simulink library "aausat3_lib"  (Simulink 8.3)
settings: Solver=ode45  StartTime=0.0  StopTime=10.0  RelTol=1e-3
undefined symbols (not defined in the file or in its folder): A_wire_mt, albedo_wrapper, alpha_0_mt, bias_gyro, bias_mag, bias_sun, Cd, coil_dim, Dim, f_sample, G, heading_gyro, heading_mag, M_earth, M_moon, M_sun, magnitude, n_mt, noise_gyro, noise_mag, noise_sun, nr_sample_sun, otoquest, otoquest_with_pro, q_method, qmethod, redfac, refldata, s_freq_gyro, s_freq_mag, s_freq_sun, sigma_0_mt, solar_absorb_coeff, solar_m_flux, SVD_method, T_0_mt, theta_e, tilt_gyro, tilt_mag, Ts
undefined symbols (not defined in the file): Actuator_Duty_Cycle_coil, Actuator_Frequency_coil, Dimensions_coil, mean_refl, Number_of_Windings_coil, rho, sim_par, svd_weigth, Wire_Cross_Sectional_Area_coil, Wire_Resistivity_Base_Temperature_coil, Wire_Resistivity_coil, Wire_Resistivity_Temperature_Coefficient_coil
libraries: aausat3_lib x118, simulink_extras x3
(part 2 of 4)

== system aausat3_lib/ADS/q-method (AAUSAT3) ==
  Sun_S : Inport  SampleTime=1
  Mag_S : Inport  Port=2  SampleTime=1
  Sun_I : Inport  Port=3  SampleTime=1
  Mag_I : Inport  Port=4  SampleTime=1
  Mux : Mux  Inputs=5
  To unit vector{,1..3} (4 alike) : aausat3_lib/Math Utilities/Vector operations/To unit vector  SystemSampleTime=-1
  Weights : Constant  Value=weigth_a
  qmethod.m : MATLABFcn  MATLABFcn=q_method([u(1) u(4);u(2) u(5);u(3) u(6)] , [u(7) u(10);u(8) u(11); u(9) u(12)], [u(13);u(14)])  OutputDimensions=4  Output1D=off
  q(I->S) : Outport  PortDimensions=4
  wires:
  Sun_I/1 -> To unit vector2/1
  Mux/1 -> qmethod.m/1
  To unit vector/1 -> Mux/1
  To unit vector2/1 -> Mux/3
  Sun_S/1 -> To unit vector/1
  Mag_I/1 -> To unit vector3/1
  To unit vector3/1 -> Mux/4
  To unit vector1/1 -> Mux/2
  Mag_S/1 -> To unit vector1/1
  Weights/1 -> Mux/5
  qmethod.m/1 -> q(I->S)/1

== system aausat3_lib/ADS/svd-method (AAUSAT3) ==
  Sun_S : Inport  SampleTime=1
  Mag_S : Inport  Port=2  SampleTime=1
  Sun_I : Inport  Port=3  SampleTime=1
  Mag_I : Inport  Port=4  SampleTime=1
  Enable : EnablePort
  Demux : Demux  Outputs=5
  Mux : Mux  Inputs=5
  Mux1 : Mux
  To unit vector{,1..3} (4 alike) : aausat3_lib/Math Utilities/Vector operations/To unit vector  SystemSampleTime=-1
  Weights : Constant  Value=weigth_a
  svd_method.m : MATLABFcn  MATLABFcn=SVD_method(u(13),[u(7);u(8);u(9)],[u(1);u(2);u(3)],u(14),[u(10);u(11);u(12)],[u(4);u(5);u(6)],0)  OutputDimensions=5  Output1D=off  SampleTime=1/f_sample
  q(I->S) : Outport  PortDimensions=4
  err : Outport  Port=2
  wires:
  Demux/5 -> err/1
  Mux1/1 -> q(I->S)/1
  svd_method.m/1 -> Demux/1
  Demux/4 -> Mux1/4
  Demux/3 -> Mux1/3
  Demux/2 -> Mux1/2
  Demux/1 -> Mux1/1
  Sun_I/1 -> To unit vector2/1
  Mux/1 -> svd_method.m/1
  To unit vector/1 -> Mux/1
  To unit vector2/1 -> Mux/3
  Sun_S/1 -> To unit vector/1
  Mag_I/1 -> To unit vector3/1
  To unit vector3/1 -> Mux/4
  To unit vector1/1 -> Mux/2
  Mag_S/1 -> To unit vector1/1
  Weights/1 -> Mux/5

== system aausat3_lib/Actuator Emulation/Magnetorquer ==
  note: m_{mt_{vec}}
  note: m_{mt}
  note: i_{mt}
  note: R_{mt}(T)
  v_mt : Inport
  coil normal : Inport  Port=2
  B(s) : Inport  Port=3
  T : Inport  Port=4
  Abs : Abs
  Area : Constant  Value=coil_dim(1)*coil_dim(2)
  Cross Product : aausat3_lib/Math Utilities/Vector operations/Cross Product
  Prodct1 : Product  Inputs=*/  RndMeth=Zero
  Prodct5 : Product  Inputs=*/  RndMeth=Zero
  Product : Product  Inputs=3  RndMeth=Zero
  Product1 : Product  Inputs=3  RndMeth=Zero
  Product2 : Product  RndMeth=Zero
  Product3 : Product  Inputs=3  RndMeth=Zero
  Product5 : Product  RndMeth=Zero
  Resistivity : Constant  Value=sigma_0_mt
  Resistivity base temperature : Constant  Value=T_0_mt
  Resistivity temperature coefficient : Constant  Value=alpha_0_mt
  Sum : Sum  Inputs=|+-
  Sum1 : Sum  Inputs=|++
  Windings : Constant  Value=n_mt
  Windings1 : Constant  Value=n_mt
  Wire cross sectional area : Constant  Value=A_wire_mt
  wire  circumference : Constant  Value=2*coil_dim(1)+2*coil_dim(2)
  N_mt(s) : Outport
  P_mt : Outport  Port=2
  m_mt_max : Outport  Port=3
  wires:
  Cross Product/1 -> N_mt(s)/1
  Product2/1 -> m_mt_max/1, Cross Product/1
  Product/1 -> Product2/2
  Area/1 -> Product/2
  Windings/1 -> Product/1
  Prodct1/1 -> Product/3, Product5/1
  coil normal/1 -> Product2/1
  Resistivity base temperature/1 -> Sum/2
  T/1 -> Sum/1
  Resistivity temperature coefficient/1 -> Product1/2
  Sum/1 -> Product1/1
  Resistivity/1 -> Product1/3, Sum1/2
  Product1/1 -> Sum1/1
  Sum1/1 -> Product3/1
  wire  circumference/1 -> Product3/2
  Windings1/1 -> Product3/3
  Product3/1 -> Prodct5/1
  Wire cross sectional area/1 -> Prodct5/2
  Prodct5/1 -> Prodct1/2
  B(s)/1 -> Cross Product/2
  v_mt/1 -> Prodct1/1, Product5/2
  Product5/1 -> Abs/1
  Abs/1 -> P_mt/1

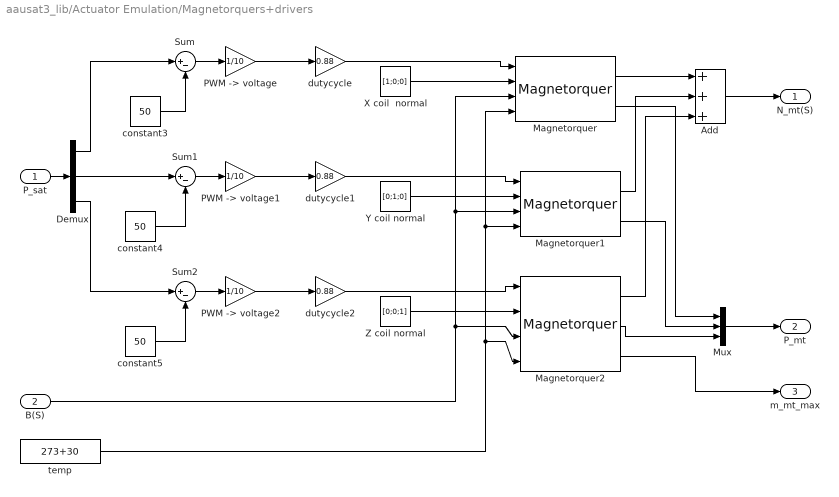
== system aausat3_lib/Actuator Emulation/Magnetorquers+drivers ==
  P_sat : Inport
  B(S) : Inport  Port=2
  Add : Sum  Inputs=+++
  Demux : Demux  Outputs=3
  Magnetorquer : aausat3_lib/Actuator Emulation/Magnetorquer  SystemSampleTime=-1  coil_dim=coil_dim  n_mt=n_mt  A_wire_mt=A_wire_mt  sigma_0_mt=sigma_0_mt  alpha_0_mt=alpha_0_mt  T_0_mt=T_0_mt
  Magnetorquer1 : aausat3_lib/Actuator Emulation/Magnetorquer  SystemSampleTime=-1  coil_dim=coil_dim  n_mt=n_mt  A_wire_mt=A_wire_mt  sigma_0_mt=sigma_0_mt  alpha_0_mt=alpha_0_mt  T_0_mt=T_0_mt
  Magnetorquer2 : aausat3_lib/Actuator Emulation/Magnetorquer  SystemSampleTime=-1  coil_dim=coil_dim  n_mt=n_mt  A_wire_mt=A_wire_mt  sigma_0_mt=sigma_0_mt  alpha_0_mt=alpha_0_mt  T_0_mt=T_0_mt
  Mux : Mux  Inputs=3
  "PWM -> voltage" : Gain  Gain=1/10
  "PWM -> voltage1" : Gain  Gain=1/10
  "PWM -> voltage2" : Gain  Gain=1/10
  Sum : Sum  Inputs=|+-
  Sum1 : Sum  Inputs=|+-
  Sum2 : Sum  Inputs=|+-
  X coil  normal : Constant  Value=[1;0;0]
  Y coil normal : Constant  Value=[0;1;0]
  Z coil normal : Constant  Value=[0;0;1]
  constant3 : Constant  Value=50
  constant4 : Constant  Value=50
  constant5 : Constant  Value=50
  dutycycle : Gain  Gain=0.88
  dutycycle1 : Gain  Gain=0.88
  dutycycle2 : Gain  Gain=0.88
  temp : Constant  Value=273+30
  N_mt(S) : Outport  PortDimensions=3
  P_mt : Outport  Port=2  PortDimensions=3
  m_mt_max : Outport  Port=3
  wires:
  Magnetorquer2/3 -> m_mt_max/1
  "PWM -> voltage2"/1 -> dutycycle2/1
  "PWM -> voltage1"/1 -> dutycycle1/1
  "PWM -> voltage"/1 -> dutycycle/1
  temp/1 -> Magnetorquer/4, Magnetorquer1/4, Magnetorquer2/4
  B(S)/1 -> Magnetorquer/3, Magnetorquer1/3, Magnetorquer2/3
  Z coil normal/1 -> Magnetorquer2/2
  Y coil normal/1 -> Magnetorquer1/2
  Magnetorquer2/1 -> Add/3
  Magnetorquer1/1 -> Add/2
  Magnetorquer/1 -> Add/1
  X coil  normal/1 -> Magnetorquer/2
  Add/1 -> N_mt(S)/1
  Magnetorquer/2 -> Mux/1
  Magnetorquer1/2 -> Mux/2
  Magnetorquer2/2 -> Mux/3
  Mux/1 -> P_mt/1
  dutycycle/1 -> Magnetorquer/1
  dutycycle1/1 -> Magnetorquer1/1
  dutycycle2/1 -> Magnetorquer2/1
  P_sat/1 -> Demux/1
  Demux/2 -> Sum1/1
  Demux/1 -> Sum/1
  Demux/3 -> Sum2/1
  Sum/1 -> "PWM -> voltage"/1
  constant3/1 -> Sum/2
  Sum1/1 -> "PWM -> voltage1"/1
  constant4/1 -> Sum1/2
  Sum2/1 -> "PWM -> voltage2"/1
  constant5/1 -> Sum2/2

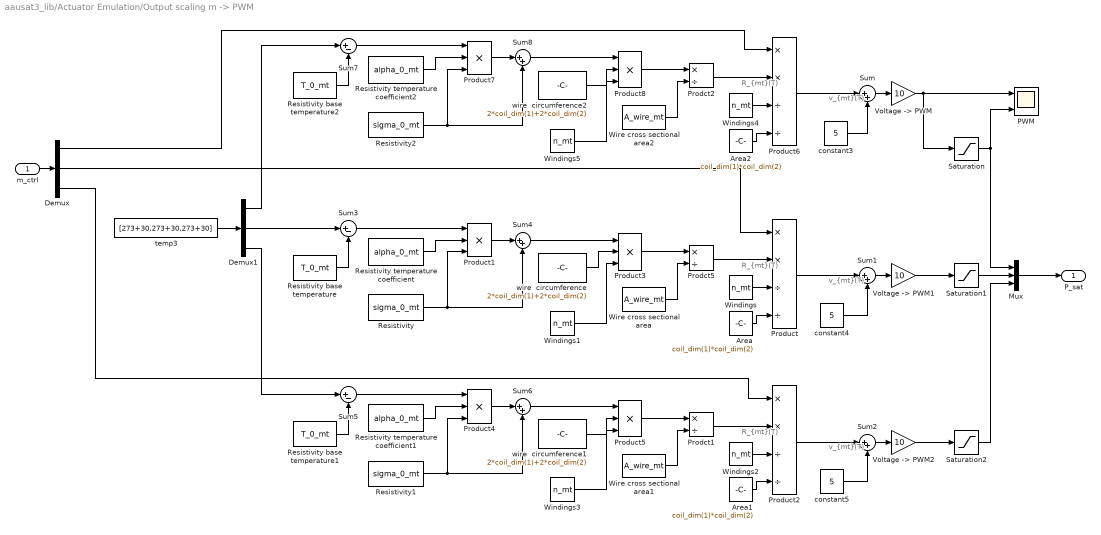
== system aausat3_lib/Actuator Emulation/Output scaling m -> PWM ==
  note: R_{mt}(T)
  note: R_{mt}(T)
  note: R_{mt}(T)
  note: v_{mt}(T)
  note: v_{mt}(T)
  note: v_{mt}(T)
  m_ctrl : Inport
  Area : Constant  Value=coil_dim(1)*coil_dim(2)
  Area1 : Constant  Value=coil_dim(1)*coil_dim(2)
  Area2 : Constant  Value=coil_dim(1)*coil_dim(2)
  Demux : Demux  Outputs=3
  Demux1 : Demux  Outputs=3
  Mux : Mux  Inputs=3
  PWM : Scope  NumInputPorts=2
      settings: TimeRange=5000  YMin=37.5~37.5  YMax=67.5~62.5  SaveName=ScopeData4  SampleInput=on
  Prodct1 : Product  Inputs=*/  RndMeth=Zero
  Prodct2 : Product  Inputs=*/  RndMeth=Zero
  Prodct5 : Product  Inputs=*/  RndMeth=Zero
  Product : Product  Inputs=**//  RndMeth=Zero
  Product{1,3..5,7..8} (6 alike) : Product  Inputs=3  RndMeth=Zero
  Product2 : Product  Inputs=**//  RndMeth=Zero
  Product6 : Product  Inputs=**//  RndMeth=Zero
  Resistivity : Constant  Value=sigma_0_mt
  Resistivity base temperature : Constant  Value=T_0_mt
  Resistivity base temperature1 : Constant  Value=T_0_mt
  Resistivity base temperature2 : Constant  Value=T_0_mt
  Resistivity temperature coefficient : Constant  Value=alpha_0_mt
  Resistivity temperature coefficient1 : Constant  Value=alpha_0_mt
  Resistivity temperature coefficient2 : Constant  Value=alpha_0_mt
  Resistivity1 : Constant  Value=sigma_0_mt
  Resistivity2 : Constant  Value=sigma_0_mt
  Saturation : Saturate  UpperLimit=PWM_max  LowerLimit=PWM_min
  Saturation1 : Saturate  UpperLimit=PWM_max  LowerLimit=PWM_min
  Saturation2 : Saturate  UpperLimit=PWM_max  LowerLimit=PWM_min
  Sum{,1..2,4,6,8} (6 alike) : Sum  Inputs=|++
  Sum3 : Sum  Inputs=|+-
  Sum5 : Sum  Inputs=|+-
  Sum7 : Sum  Inputs=|+-
  "Voltage -> PWM" : Gain  Gain=10
  "Voltage -> PWM1" : Gain  Gain=10
  "Voltage -> PWM2" : Gain  Gain=10
  Windings{,1..5} (6 alike) : Constant  Value=n_mt
  Wire cross sectional area : Constant  Value=A_wire_mt
  Wire cross sectional area1 : Constant  Value=A_wire_mt
  Wire cross sectional area2 : Constant  Value=A_wire_mt
  constant3 : Constant  Value=5
  constant4 : Constant  Value=5
  constant5 : Constant  Value=5
  temp3 : Constant  Value=[273+30,273+30,273+30]
  wire  circumference : Constant  Value=2*coil_dim(1)+2*coil_dim(2)
  wire  circumference1 : Constant  Value=2*coil_dim(1)+2*coil_dim(2)
  wire  circumference2 : Constant  Value=2*coil_dim(1)+2*coil_dim(2)
  P_sat : Outport  PortDimensions=3
  wires:
  Prodct2/1 -> Product6/2
  Prodct5/1 -> Product/2
  Prodct1/1 -> Product2/2
  Resistivity base temperature2/1 -> Sum7/2
  Resistivity temperature coefficient2/1 -> Product7/2
  Sum7/1 -> Product7/1
  Resistivity2/1 -> Product7/3, Sum8/2
  Product7/1 -> Sum8/1
  Sum8/1 -> Product8/1
  wire  circumference2/1 -> Product8/2
  Windings5/1 -> Product8/3
  Product8/1 -> Prodct2/1
  Wire cross sectional area2/1 -> Prodct2/2
  Demux1/1 -> Sum7/1
  Resistivity base temperature/1 -> Sum3/2
  Resistivity temperature coefficient/1 -> Product1/2
  Sum3/1 -> Product1/1
  Resistivity/1 -> Product1/3, Sum4/2
  Product1/1 -> Sum4/1
  Sum4/1 -> Product3/1
  wire  circumference/1 -> Product3/2
  Windings1/1 -> Product3/3
  Product3/1 -> Prodct5/1
  Wire cross sectional area/1 -> Prodct5/2
  Demux1/2 -> Sum3/1
  Demux1/3 -> Sum5/1
  Resistivity base temperature1/1 -> Sum5/2
  Resistivity temperature coefficient1/1 -> Product4/2
  Sum5/1 -> Product4/1
  Resistivity1/1 -> Product4/3, Sum6/2
  Product4/1 -> Sum6/1
  Sum6/1 -> Product5/1
  wire  circumference1/1 -> Product5/2
  Windings3/1 -> Product5/3
  Product5/1 -> Prodct1/1
  Wire cross sectional area1/1 -> Prodct1/2
  constant5/1 -> Sum2/2
  constant4/1 -> Sum1/2
  constant3/1 -> Sum/2
  m_ctrl/1 -> Demux/1
  Mux/1 -> P_sat/1
  Saturation/1 -> PWM/2, Mux/1
  Saturation1/1 -> Mux/2
  Saturation2/1 -> Mux/3
  Sum/1 -> "Voltage -> PWM"/1
  Sum1/1 -> "Voltage -> PWM1"/1
  Sum2/1 -> "Voltage -> PWM2"/1
  temp3/1 -> Demux1/1
  Windings/1 -> Product/3
  Area/1 -> Product/4
  Windings2/1 -> Product2/3
  Area1/1 -> Product2/4
  Windings4/1 -> Product6/3
  Area2/1 -> Product6/4
  "Voltage -> PWM"/1 -> PWM/1, Saturation/1
  "Voltage -> PWM1"/1 -> Saturation1/1
  "Voltage -> PWM2"/1 -> Saturation2/1
  Demux/1 -> Product6/1
  Demux/2 -> Product/1
  Demux/3 -> Product2/1
  Product6/1 -> Sum/1
  Product/1 -> Sum1/1
  Product2/1 -> Sum2/1

== system aausat3_lib/Actuator Emulation/Permanent Magnet ==
  Attitude q(I->S) : Inport
  Magnetic field B(I) : Inport  Port=2
  Enable : EnablePort
  Cross Product : aausat3_lib/Math Utilities/Vector operations/Cross Product  SystemSampleTime=-1
  Magnetic dipole moment : Constant  Value=[0,0,mag_moment]
  Vector rotation by q : Subsystem
  N_mpmag(S) : Outport
  wires:
  Magnetic dipole moment/1 -> Cross Product/1
  Vector rotation by q/1(q'Vq) -> Cross Product/2
  Cross Product/1 -> N_mpmag(S)/1
  Attitude q(I->S)/1 -> Vector rotation by q/1(q)
  Magnetic field B(I)/1 -> Vector rotation by q/2(V)

== system aausat3_lib/Disturbances/Atmospheric ==
  q(I->S) : Inport
  V_sc(I) : Inport  Port=2
  R_com(S) : Inport  Port=3
  inclination : Inport  Port=4
  r_pos : Inport  Port=5
  jd : Inport  Port=6
  Enable : EnablePort
  C_D1 : Constant  Value=Cd
  Demux : Demux  Outputs=6
  Density7 : Subsystem
  MATLAB Function : MATLAB Function  TreatAsAtomicUnit=on
  Mux : Mux  Inputs=6
  Mux1 : Mux  Inputs=3
  Mux2 : Mux  Inputs=3
  N_atm(S) : Outport
  F_atm(I) : Outport  Port=2
  wires:
  Mux/1 -> MATLAB Function/1(input)
  MATLAB Function/1(out) -> Demux/1
  Demux/3 -> Mux1/3
  Demux/2 -> Mux1/2
  Demux/1 -> Mux1/1
  Demux/6 -> Mux2/3
  Demux/5 -> Mux2/2
  Demux/4 -> Mux2/1
  Mux2/1 -> F_atm(I)/1
  Mux1/1 -> N_atm(S)/1
  q(I->S)/1 -> Mux/6
  V_sc(I)/1 -> Mux/4
  C_D1/1 -> Mux/2
  jd/1 -> Density7/3(jd)
  inclination/1 -> Density7/1(i)
  r_pos/1 -> Density7/2(r), Mux/5
  Density7/1(rho) -> Mux/1
  R_com(S)/1 -> Mux/3  "Center of Mass"

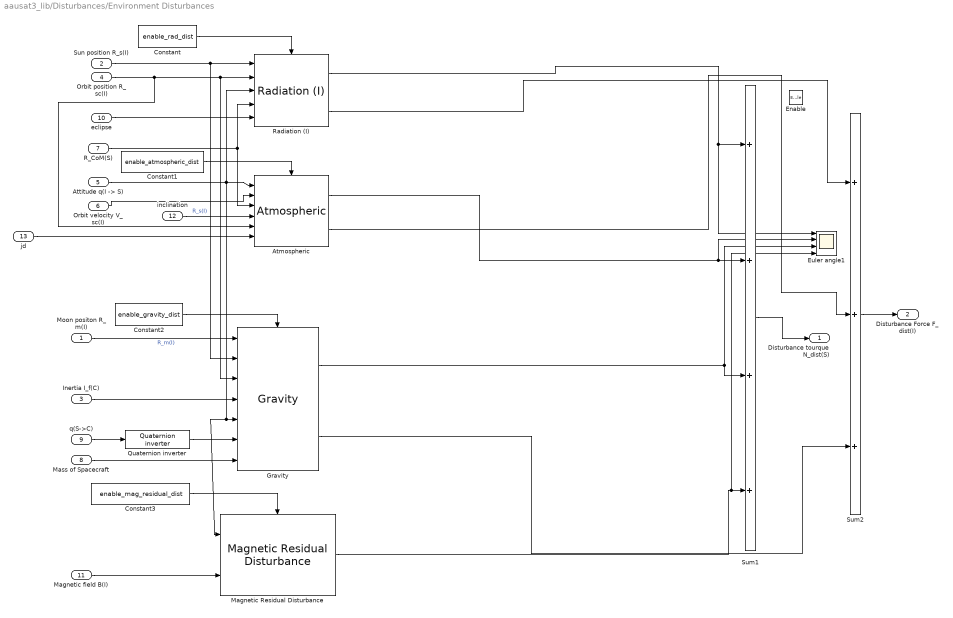
== system aausat3_lib/Disturbances/Environment Disturbances ==
  Moon positon R_m(I) : Inport
  Sun position R_s(I) : Inport  Port=2
  Inertia I_f(C) : Inport  Port=3
  Orbit position R_sc(I) : Inport  Port=4
  "Attitude q(I -> S)" : Inport  Port=5
  Orbit velocity V_sc(I) : Inport  Port=6
  R_CoM(S) : Inport  Port=7
  Mass of Spacecraft : Inport  Port=8
  q(S->C) : Inport  Port=9
  eclipse : Inport  Port=10
  Magnetic field B(I) : Inport  Port=11
  inclination : Inport  Port=12
  jd : Inport  Port=13
  Enable : EnablePort
  Atmospheric : aausat3_lib/Disturbances/Atmospheric  Cd=Cd  rho=rho
  Constant : Constant  Value=enable_rad_dist
  Constant1 : Constant  Value=enable_atmospheric_dist
  Constant2 : Constant  Value=enable_gravity_dist
  Constant3 : Constant  Value=enable_mag_residual_dist
  Euler angle1 : Scope  NumInputPorts=4
      settings: TimeRange=5000  YMin=-2e-08~-4e-07~-1.5e-08~-4e-08  YMax=2e-08~4e-07~1.5e-08~4e-08  SaveName=dist_sep  SampleInput=on
  Gravity : aausat3_lib/Disturbances/Gravity  G=G  M_sun=M_sun  M_moon=M_moon  M_earth=M_earth  enable_moon_G=on  enable_sun_G=on  enable_zharm_earth=on  enable_gravity_torque=on
  Magnetic Residual Disturbance : aausat3_lib/Disturbances/Magnetic Residual Disturbance  mag_moment=0.00033
  Quaternion inverter : aausat3_lib/Math Utilities/Quaternion operations/Quaternion inverter
  Radiation (I) : aausat3_lib/Disturbances/Radiation (I)  Dim=Dim  solar_m_flux=solar_m_flux  solar_absorb_coeff=solar_absorb_coeff
  Sum1 : Sum  Inputs=++++  SaturateOnIntegerOverflow=on
  Sum2 : Sum  Inputs=+++  SaturateOnIntegerOverflow=on
  Disturbance tourque N_dist(S) : Outport
  Disturbance Force F_dist(I) : Outport  Port=2
  wires:
  jd/1 -> Atmospheric/6
  inclination/1 -> Atmospheric/4
  Sum2/1 -> Disturbance Force F_dist(I)/1
  Radiation (I)/1 -> Euler angle1/1, Sum1/1
  Atmospheric/1 -> Euler angle1/2, Sum1/2
  Gravity/1 -> Euler angle1/3, Sum1/3
  Magnetic Residual Disturbance/1 -> Euler angle1/4, Sum1/4
  Atmospheric/2 -> Sum2/2
  Inertia I_f(C)/1 -> Gravity/4
  eclipse/1 -> Radiation (I)/5
  Sum1/1 -> Disturbance tourque N_dist(S)/1
  Gravity/2 -> Sum2/3
  Radiation (I)/2 -> Sum2/1
  Orbit velocity V_sc(I)/1 -> Atmospheric/2
  Orbit position R_sc(I)/1 -> Radiation (I)/2, Gravity/3, Atmospheric/5
  "Attitude q(I -> S)"/1 -> Radiation (I)/3, Atmospheric/1, Gravity/5, Magnetic Residual Disturbance/1
  Sun position R_s(I)/1 -> Radiation (I)/1, Gravity/2  "R_s(I)"
  Moon positon R_m(I)/1 -> Gravity/1  "R_m(I)"
  Mass of Spacecraft/1 -> Gravity/7
  Quaternion inverter/1 -> Gravity/6
  q(S->C)/1 -> Quaternion inverter/1
  R_CoM(S)/1 -> Radiation (I)/4, Atmospheric/3
  Constant/1 -> Radiation (I)/Enable
  Constant2/1 -> Gravity/Enable
  Constant1/1 -> Atmospheric/Enable
  Constant3/1 -> Magnetic Residual Disturbance/Enable
  Magnetic field B(I)/1 -> Magnetic Residual Disturbance/2

== system aausat3_lib/Disturbances/Gravity ==
  R_m(I) : Inport
  R_s(I) : Inport  Port=2
  R_sc(I) : Inport  Port=3
  I(C) : Inport  Port=4
  "q(I -> S)" : Inport  Port=5
  q(C->S) : Inport  Port=6
  M_sat : Inport  Port=7
  Enable : EnablePort
  Constant : Constant  Value=enable_moon_G
  Constant1 : Constant  Value=enable_sun_G
  Constant2 : Constant  Value=enable_zharm_earth
  Constant3 : Constant  Value=enable_gravity_torque
  Gravity Gradient Torque : aausat3_lib/Disturbances/Gravity Gradient Torque  G=G  M_earth=M_earth
  Gravity Moon : aausat3_lib/Disturbances/Gravity Moon  G=G  M_moon=M_moon
  Gravity Sun : aausat3_lib/Disturbances/Gravity Sun  G=G  M_sun=M_sun
  Sum : Sum  Inputs=++++  SaturateOnIntegerOverflow=on
  Sum1 : Sum  Inputs=|+-  SaturateOnIntegerOverflow=on
  Sum2 : Sum  Inputs=|+-  SaturateOnIntegerOverflow=on
  Sum3 : Sum  Inputs=++++  SaturateOnIntegerOverflow=on
  Zonal Harmonics  Earth : aausat3_lib/Disturbances/Zonal Harmonics  Earth
  N_gr(S) : Outport
  F_gr(I) : Outport  Port=2
  wires:
  Zonal Harmonics  Earth/2 -> Sum3/3
  Gravity Sun/2 -> Sum3/2
  Gravity Moon/2 -> Sum3/1
  Sum3/1 -> N_gr(S)/1
  I(C)/1 -> Zonal Harmonics  Earth/3, Gravity Sun/2, Gravity Moon/2, Gravity Gradient Torque/2
  q(C->S)/1 -> Zonal Harmonics  Earth/4, Gravity Sun/3, Gravity Moon/3, Gravity Gradient Torque/3
  "q(I -> S)"/1 -> Zonal Harmonics  Earth/5, Gravity Gradient Torque/4, Gravity Sun/4, Gravity Moon/4
  M_sat/1 -> Gravity Sun/1, Zonal Harmonics  Earth/1, Gravity Moon/1, Gravity Gradient Torque/5
  Sum/1 -> F_gr(I)/1
  Zonal Harmonics  Earth/1 -> Sum/3
  R_m(I)/1 -> Sum1/1
  R_s(I)/1 -> Sum2/1
  Gravity Moon/1 -> Sum/1
  Gravity Sun/1 -> Sum/2
  Constant3/1 -> Gravity Gradient Torque/Enable
  Constant2/1 -> Zonal Harmonics  Earth/Enable
  Constant1/1 -> Gravity Sun/Enable
  Constant/1 -> Gravity Moon/Enable
  R_sc(I)/1 -> Sum1/2, Sum2/2, Zonal Harmonics  Earth/2, Gravity Gradient Torque/1
  Sum2/1 -> Gravity Sun/5
  Sum1/1 -> Gravity Moon/5
  Gravity Gradient Torque/1 -> Sum3/4
  Gravity Gradient Torque/2 -> Sum/4

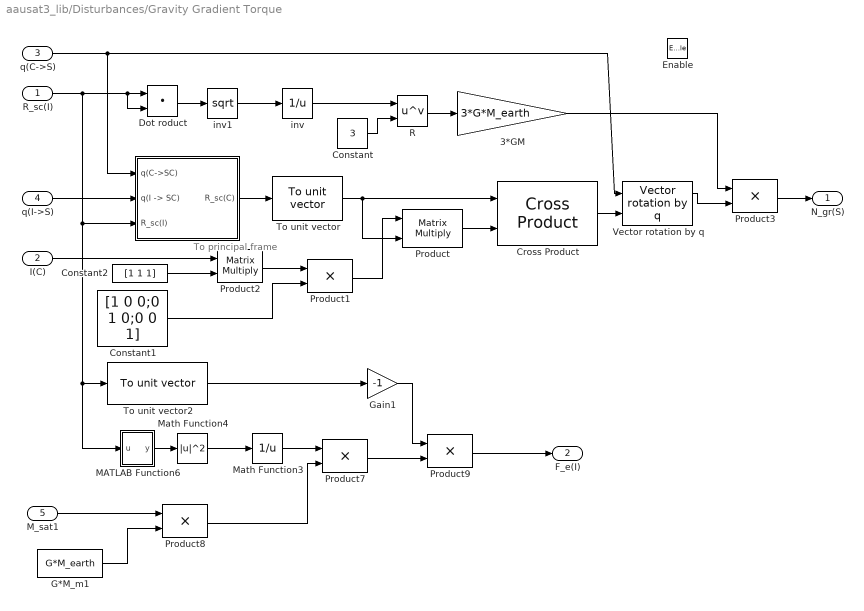
== system aausat3_lib/Disturbances/Gravity Gradient Torque ==
  note: To principal frame
  R_sc(I) : Inport
  I(C) : Inport  Port=2
  q(C->S) : Inport  Port=3
  q(I->S) : Inport  Port=4
  M_sat1 : Inport  Port=5
  Enable : EnablePort
  " " : Subsystem
  3*GM : Gain  Gain=3*G*M_earth  SaturateOnIntegerOverflow=on  OutDataTypeStr=Inherit: Same as input  ParamDataTypeStr=Inherit: Same as input
  Constant : Constant  Value=3
  Constant1 : Constant  Value=[1 0 0;0 1 0;0 0 1]
  Constant2 : Constant  Value=[1 1 1]  VectorParams1D=off
  Cross Product : aausat3_lib/Math Utilities/Vector operations/Cross Product
  Dot roduct : DotProduct  InputSameDT=on  OutDataTypeStr=Inherit: Inherit via internal rule
  G*M_m1 : Constant  Value=G*M_earth
  Gain1 : Gain  Gain=-1  SaturateOnIntegerOverflow=on  OutDataTypeStr=Inherit: Same as input  ParamDataTypeStr=Inherit: Same as input
  MATLAB Function6 : MATLAB Function  TreatAsAtomicUnit=on
  Math Function3 : Math  Operator=reciprocal  SaturateOnIntegerOverflow=on
  Math Function4 : Math  Operator=magnitude^2  SaturateOnIntegerOverflow=on
  Product : Product  Multiplication=Matrix(*)  SaturateOnIntegerOverflow=on  OutDataTypeStr=Inherit: Same as first input
  Product{1,3,7..9} (5 alike) : Product  SaturateOnIntegerOverflow=on  OutDataTypeStr=Inherit: Same as first input
  Product2 : Product  Multiplication=Matrix(*)  SaturateOnIntegerOverflow=on  OutDataTypeStr=Inherit: Same as first input
  R : Math  Operator=pow  SaturateOnIntegerOverflow=on
  To unit vector : aausat3_lib/Math Utilities/Vector operations/To unit vector
  To unit vector2 : aausat3_lib/Math Utilities/Vector operations/To unit vector
  Vector rotation by q : aausat3_lib/Math Utilities/Quaternion operations/Vector rotation by q
  inv : Math  Operator=reciprocal  SaturateOnIntegerOverflow=on
  inv1 : Math  Operator=sqrt  SaturateOnIntegerOverflow=on
  N_gr(S) : Outport
  F_e(I) : Outport  Port=2
  wires:
  MATLAB Function6/1(y) -> Math Function4/1
  Cross Product/1 -> Vector rotation by q/2
  Dot roduct/1 -> inv1/1
  Product3/1 -> N_gr(S)/1
  R/1 -> 3*GM/1
  inv/1 -> R/1
  inv1/1 -> inv/1
  Constant/1 -> R/2
  To unit vector/1 -> Product/2, Cross Product/1
  q(C->S)/1 -> " "/1(q(C->SC)), Vector rotation by q/1
  q(I->S)/1 -> " "/2("q(I -> SC)")
  " "/1(R_sc(C)) -> To unit vector/1
  Product1/1 -> Product/1
  Product/1 -> Cross Product/2
  I(C)/1 -> Product2/1
  Constant2/1 -> Product2/2
  Product2/1 -> Product1/1
  Constant1/1 -> Product1/2
  R_sc(I)/1 -> Dot roduct/2, Dot roduct/1, " "/3(R_sc(I)), To unit vector2/1, MATLAB Function6/1(u)
  3*GM/1 -> Product3/1
  Vector rotation by q/1 -> Product3/2
  Math Function4/1 -> Math Function3/1
  M_sat1/1 -> Product8/1
  G*M_m1/1 -> Product8/2
  Math Function3/1 -> Product7/1
  Product8/1 -> Product7/2
  To unit vector2/1 -> Gain1/1
  Product9/1 -> F_e(I)/1
  Gain1/1 -> Product9/1
  Product7/1 -> Product9/2

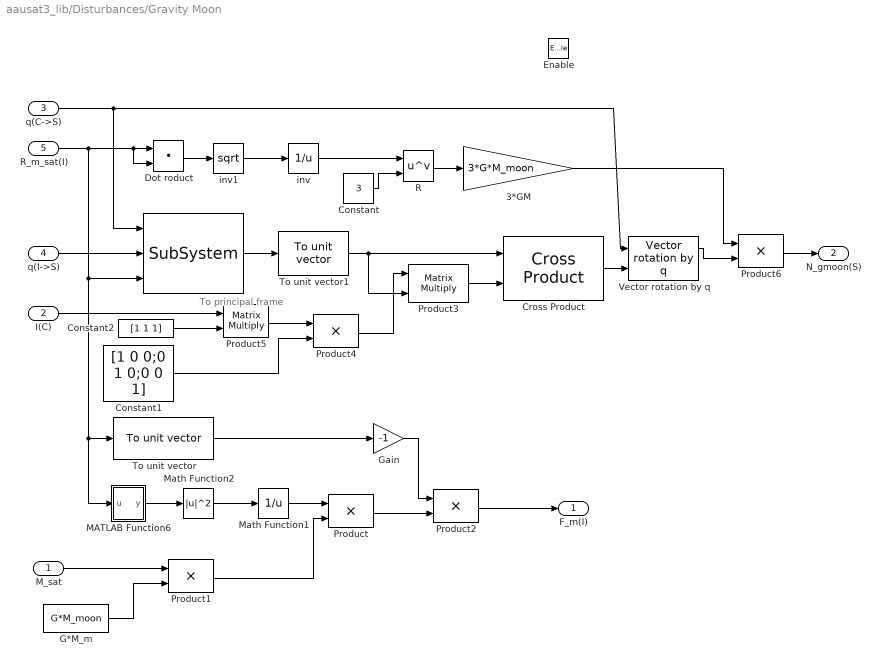
== system aausat3_lib/Disturbances/Gravity Moon ==
  note: To principal frame
  M_sat : Inport
  I(C) : Inport  Port=2
  q(C->S) : Inport  Port=3
  q(I->S) : Inport  Port=4
  R_m_sat(I) : Inport  Port=5
  Enable : EnablePort
  " " : aausat3_lib/Disturbances/Gravity Gradient Torque/ 
  3*GM : Gain  Gain=3*G*M_moon  SaturateOnIntegerOverflow=on  OutDataTypeStr=Inherit: Same as input  ParamDataTypeStr=Inherit: Same as input
  Constant : Constant  Value=3
  Constant1 : Constant  Value=[1 0 0;0 1 0;0 0 1]
  Constant2 : Constant  Value=[1 1 1]  VectorParams1D=off
  Cross Product : aausat3_lib/Math Utilities/Vector operations/Cross Product
  Dot roduct : DotProduct  InputSameDT=on  OutDataTypeStr=Inherit: Inherit via internal rule
  G*M_m : Constant  Value=G*M_moon
  Gain : Gain  Gain=-1  SaturateOnIntegerOverflow=on  OutDataTypeStr=Inherit: Same as input  ParamDataTypeStr=Inherit: Same as input
  MATLAB Function6 : MATLAB Function  TreatAsAtomicUnit=on
  Math Function1 : Math  Operator=reciprocal  SaturateOnIntegerOverflow=on
  Math Function2 : Math  Operator=magnitude^2  SaturateOnIntegerOverflow=on
  Product{,1..2,4,6} (5 alike) : Product  SaturateOnIntegerOverflow=on  OutDataTypeStr=Inherit: Same as first input
  Product3 : Product  Multiplication=Matrix(*)  SaturateOnIntegerOverflow=on  OutDataTypeStr=Inherit: Same as first input
  Product5 : Product  Multiplication=Matrix(*)  SaturateOnIntegerOverflow=on  OutDataTypeStr=Inherit: Same as first input
  R : Math  Operator=pow  SaturateOnIntegerOverflow=on
  To unit vector : aausat3_lib/Math Utilities/Vector operations/To unit vector
  To unit vector1 : aausat3_lib/Math Utilities/Vector operations/To unit vector
  Vector rotation by q : aausat3_lib/Math Utilities/Quaternion operations/Vector rotation by q
  inv : Math  Operator=reciprocal  SaturateOnIntegerOverflow=on
  inv1 : Math  Operator=sqrt  SaturateOnIntegerOverflow=on
  F_m(I) : Outport
  N_gmoon(S) : Outport  Port=2
  wires:
  MATLAB Function6/1(y) -> Math Function2/1
  Math Function2/1 -> Math Function1/1
  M_sat/1 -> Product1/1
  G*M_m/1 -> Product1/2
  Math Function1/1 -> Product/1
  Product1/1 -> Product/2
  To unit vector/1 -> Gain/1
  Product2/1 -> F_m(I)/1
  Gain/1 -> Product2/1
  Product/1 -> Product2/2
  Vector rotation by q/1 -> Product6/2
  3*GM/1 -> Product6/1
  Constant1/1 -> Product4/2
  Product5/1 -> Product4/1
  Constant2/1 -> Product5/2
  I(C)/1 -> Product5/1
  Product3/1 -> Cross Product/2
  Product4/1 -> Product3/1
  " "/1 -> To unit vector1/1
  q(I->S)/1 -> " "/2
  q(C->S)/1 -> Vector rotation by q/1, " "/1
  To unit vector1/1 -> Cross Product/1, Product3/2
  Constant/1 -> R/2
  inv1/1 -> inv/1
  inv/1 -> R/1
  R/1 -> 3*GM/1
  Product6/1 -> N_gmoon(S)/1
  Dot roduct/1 -> inv1/1
  Cross Product/1 -> Vector rotation by q/2
  R_m_sat(I)/1 -> Dot roduct/1, Dot roduct/2, " "/3, To unit vector/1, MATLAB Function6/1(u)

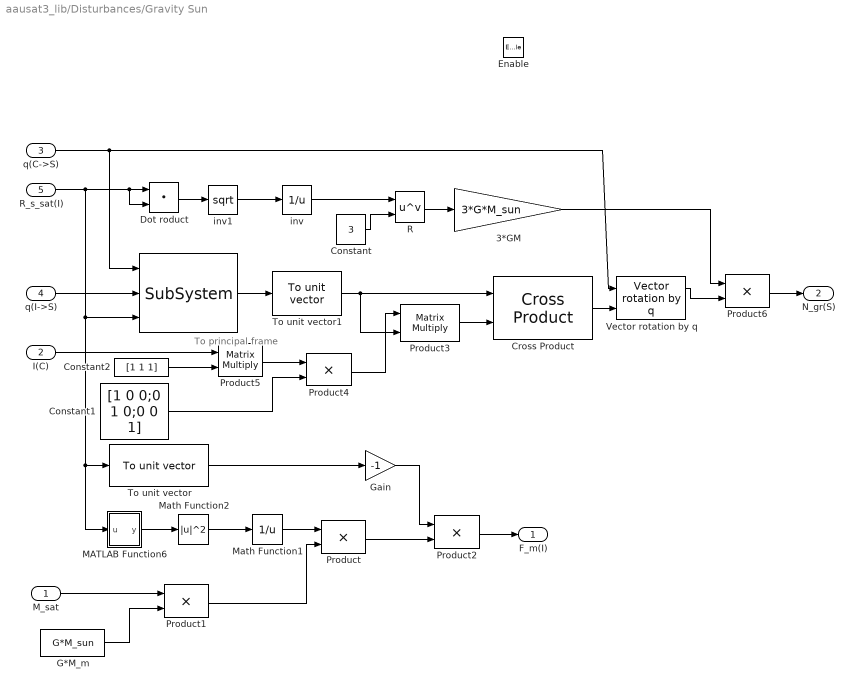
== system aausat3_lib/Disturbances/Gravity Sun ==
  note: To principal frame
  M_sat : Inport
  I(C) : Inport  Port=2
  q(C->S) : Inport  Port=3
  q(I->S) : Inport  Port=4
  R_s_sat(I) : Inport  Port=5
  Enable : EnablePort
  " " : aausat3_lib/Disturbances/Gravity Gradient Torque/ 
  3*GM : Gain  Gain=3*G*M_sun  SaturateOnIntegerOverflow=on  OutDataTypeStr=Inherit: Same as input  ParamDataTypeStr=Inherit: Same as input
  Constant : Constant  Value=3
  Constant1 : Constant  Value=[1 0 0;0 1 0;0 0 1]
  Constant2 : Constant  Value=[1 1 1]  VectorParams1D=off
  Cross Product : aausat3_lib/Math Utilities/Vector operations/Cross Product
  Dot roduct : DotProduct  InputSameDT=on  OutDataTypeStr=Inherit: Inherit via internal rule
  G*M_m : Constant  Value=G*M_sun
  Gain : Gain  Gain=-1  SaturateOnIntegerOverflow=on  OutDataTypeStr=Inherit: Same as input  ParamDataTypeStr=Inherit: Same as input
  MATLAB Function6 : MATLAB Function  TreatAsAtomicUnit=on
  Math Function1 : Math  Operator=reciprocal  SaturateOnIntegerOverflow=on
  Math Function2 : Math  Operator=magnitude^2  SaturateOnIntegerOverflow=on
  Product{,1..2,4,6} (5 alike) : Product  SaturateOnIntegerOverflow=on  OutDataTypeStr=Inherit: Same as first input
  Product3 : Product  Multiplication=Matrix(*)  SaturateOnIntegerOverflow=on  OutDataTypeStr=Inherit: Same as first input
  Product5 : Product  Multiplication=Matrix(*)  SaturateOnIntegerOverflow=on  OutDataTypeStr=Inherit: Same as first input
  R : Math  Operator=pow  SaturateOnIntegerOverflow=on
  To unit vector : aausat3_lib/Math Utilities/Vector operations/To unit vector
  To unit vector1 : aausat3_lib/Math Utilities/Vector operations/To unit vector
  Vector rotation by q : aausat3_lib/Math Utilities/Quaternion operations/Vector rotation by q
  inv : Math  Operator=reciprocal  SaturateOnIntegerOverflow=on
  inv1 : Math  Operator=sqrt  SaturateOnIntegerOverflow=on
  F_m(I) : Outport
  N_gr(S) : Outport  Port=2
  wires:
  MATLAB Function6/1(y) -> Math Function2/1
  Product/1 -> Product2/2
  Gain/1 -> Product2/1
  Product2/1 -> F_m(I)/1
  To unit vector/1 -> Gain/1
  Product1/1 -> Product/2
  Math Function1/1 -> Product/1
  G*M_m/1 -> Product1/2
  M_sat/1 -> Product1/1
  Math Function2/1 -> Math Function1/1
  Vector rotation by q/1 -> Product6/2
  3*GM/1 -> Product6/1
  R_s_sat(I)/1 -> Dot roduct/1, Dot roduct/2, " "/3, To unit vector/1, MATLAB Function6/1(u)
  Constant1/1 -> Product4/2
  Product5/1 -> Product4/1
  Constant2/1 -> Product5/2
  I(C)/1 -> Product5/1
  Product3/1 -> Cross Product/2
  Product4/1 -> Product3/1
  " "/1 -> To unit vector1/1
  q(I->S)/1 -> " "/2
  q(C->S)/1 -> Vector rotation by q/1, " "/1
  To unit vector1/1 -> Cross Product/1, Product3/2
  Constant/1 -> R/2
  inv1/1 -> inv/1
  inv/1 -> R/1
  R/1 -> 3*GM/1
  Product6/1 -> N_gr(S)/1
  Dot roduct/1 -> inv1/1
  Cross Product/1 -> Vector rotation by q/2

== system aausat3_lib/Disturbances/Magnetic Residual Disturbance ==
  Attitude q(I->S) : Inport
  Magnetic field B(I) : Inport  Port=2
  Enable : EnablePort
  Cross Product : aausat3_lib/Math Utilities/Vector operations/Cross Product
  Product : Product  RndMeth=Zero
  Random Number : RandomNumber  Variance=mag_moment^2  Seed=23751
  Randome 3D Vector : aausat3_lib/Other Model Utilities/Randome 3D Vector  mean=0  var=100  seed=[23314,67594,99812]
  Vector rotation by q : aausat3_lib/Math Utilities/Quaternion operations/Vector rotation by q
  N_mres(S) : Outport
  wires:
  Cross Product/1 -> N_mres(S)/1
  Random Number/1 -> Product/1
  Product/1 -> Cross Product/1
  Randome 3D Vector/1 -> Product/2
  Magnetic field B(I)/1 -> Vector rotation by q/2
  Attitude q(I->S)/1 -> Vector rotation by q/1
  Vector rotation by q/1 -> Cross Product/2

== system aausat3_lib/Disturbances/Radiation (I) ==
  note: Radiation force
  note: Earth rotation
  note: Sun line
  R_s(I) : Inport
  R_sat(I) : Inport  Port=2
  q(I->S) : Inport  Port=3
  R_com(S) : Inport  Port=4
  eclipse : Inport  Port=5
  Enable : EnablePort
  Absorbtion Coefficient : Constant  Value=solar_absorb_coeff
  Absorbtion Coefficient1 : Constant  Value=[0;0;0]
  Cross Product : aausat3_lib/Math Utilities/Vector operations/Cross Product
  Dimensions : Constant  Value=Dim
  Exposed area : aausat3_lib/Other Model Utilities/Exposed area  dim_sat_area=Dim
  Gain : Gain  Gain=-1  SaturateOnIntegerOverflow=on  OutDataTypeStr=Inherit: Same as input  ParamDataTypeStr=Inherit: Same as input
  Gain1 : Gain  Gain=1/2  SaturateOnIntegerOverflow=on  OutDataTypeStr=Inherit: Same as input  ParamDataTypeStr=Inherit: Same as input
  Momentum flux from the sun : Constant  Value=solar_m_flux
  Product1 : Product  SaturateOnIntegerOverflow=on  OutDataTypeStr=Inherit: Same as first input
  Product2 : Product  SaturateOnIntegerOverflow=on  OutDataTypeStr=Inherit: Same as first input
  Product4 : Product  SaturateOnIntegerOverflow=on  OutDataTypeStr=Inherit: Same as first input
  Sum : Sum  Inputs=|+-  SaturateOnIntegerOverflow=on
  Sum1 : Sum  Inputs=|+-
  Switch : Switch  Criteria=u2 ~= 0
  To unit vector : aausat3_lib/Math Utilities/Vector operations/To unit vector
  Vector rotation by q : aausat3_lib/Math Utilities/Quaternion operations/Vector rotation by q
  N_rad(S) : Outport
  F_rad(I) : Outport  Port=2
  wires:
  Sum1/1 -> Cross Product/1
  Gain1/1 -> Sum1/2
  R_com(S)/1 -> Sum1/1
  Dimensions/1 -> Gain1/1
  eclipse/1 -> Switch/2
  Cross Product/1 -> Switch/3
  Momentum flux from the sun/1 -> Product1/1
  Exposed area/1 -> Product1/2
  Vector rotation by q/1 -> Cross Product/2
  Gain/1 -> F_rad(I)/1, Vector rotation by q/2
  Product4/1 -> Gain/1
  To unit vector/1 -> Product4/2
  Product2/1 -> Product4/1
  Absorbtion Coefficient/1 -> Product2/2
  Product1/1 -> Product2/1
  Sum/1 -> To unit vector/1, Exposed area/2
  q(I->S)/1 -> Vector rotation by q/1, Exposed area/1
  R_sat(I)/1 -> Sum/2
  R_s(I)/1 -> Sum/1
  Switch/1 -> N_rad(S)/1
  Absorbtion Coefficient1/1 -> Switch/1

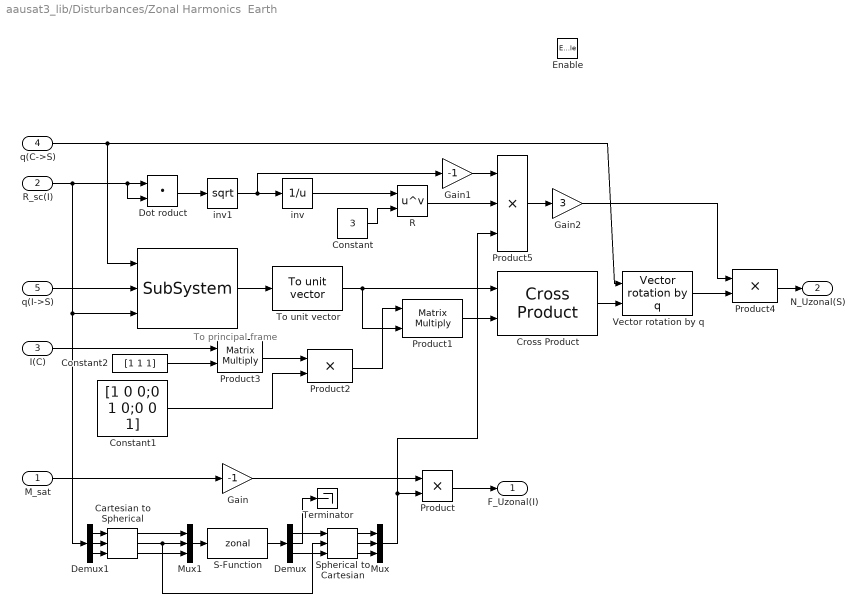
== system aausat3_lib/Disturbances/Zonal Harmonics  Earth ==
  note: To principal frame
  M_sat : Inport
  R_sc(I) : Inport  Port=2
  I(C) : Inport  Port=3
  q(C->S) : Inport  Port=4
  q(I->S) : Inport  Port=5
  Enable : EnablePort
  " " : aausat3_lib/Disturbances/Gravity Gradient Torque/   SystemSampleTime=-1
  Cartesian to Spherical : simulink_extras/Transformations/Cartesian to Spherical  SystemSampleTime=-1
  Constant : Constant  Value=3
  Constant1 : Constant  Value=[1 0 0;0 1 0;0 0 1]
  Constant2 : Constant  Value=[1 1 1]  VectorParams1D=off
  Cross Product : aausat3_lib/Math Utilities/Vector operations/Cross Product  SystemSampleTime=-1
  Demux : Demux  Outputs=3
  Demux1 : Demux  Outputs=3
  Dot roduct : DotProduct  InputSameDT=on  OutDataTypeStr=Inherit: Inherit via internal rule
  Gain : Gain  Gain=-1
  Gain1 : Gain  Gain=-1
  Gain2 : Gain  Gain=3
  Mux : Mux  Inputs=3
  Mux1 : Mux  Inputs=3
  Product : Product  RndMeth=Zero
  Product1 : Product  Multiplication=Matrix(*)  SaturateOnIntegerOverflow=on  OutDataTypeStr=Inherit: Same as first input
  Product2 : Product  SaturateOnIntegerOverflow=on  OutDataTypeStr=Inherit: Same as first input
  Product3 : Product  Multiplication=Matrix(*)  SaturateOnIntegerOverflow=on  OutDataTypeStr=Inherit: Same as first input
  Product4 : Product  SaturateOnIntegerOverflow=on  OutDataTypeStr=Inherit: Same as first input
  Product5 : Product  Inputs=3  RndMeth=Zero
  R : Math  Operator=pow  SaturateOnIntegerOverflow=on
  S-Function : S-Function  FunctionName=zonal  EnableBusSupport=off
  Spherical to Cartesian : simulink_extras/Transformations/Spherical to Cartesian  SystemSampleTime=-1
  Terminator : Terminator
  To unit vector : aausat3_lib/Math Utilities/Vector operations/To unit vector  SystemSampleTime=-1
  Vector rotation by q : aausat3_lib/Math Utilities/Quaternion operations/Vector rotation by q  SystemSampleTime=-1
  inv : Math  Operator=reciprocal  SaturateOnIntegerOverflow=on
  inv1 : Math  Operator=sqrt  SaturateOnIntegerOverflow=on
  F_Uzonal(I) : Outport
  N_Uzonal(S) : Outport  Port=2
  wires:
  Demux1/1 -> Cartesian to Spherical/1
  Demux1/2 -> Cartesian to Spherical/2
  Demux1/3 -> Cartesian to Spherical/3
  Spherical to Cartesian/1 -> Mux/1
  Spherical to Cartesian/3 -> Mux/3
  Demux/1 -> Spherical to Cartesian/1
  Demux/3 -> Spherical to Cartesian/3
  S-Function/1 -> Demux/1
  Mux1/1 -> S-Function/1
  Cartesian to Spherical/1 -> Mux1/1
  Cartesian to Spherical/3 -> Mux1/3
  Cartesian to Spherical/2 -> Mux1/2, Spherical to Cartesian/2
  Spherical to Cartesian/2 -> Mux/2
  Demux/2 -> Terminator/1
  Mux/1 -> Product/2, Product5/3
  Gain/1 -> Product/1
  M_sat/1 -> Gain/1
  Product/1 -> F_Uzonal(I)/1
  Cross Product/1 -> Vector rotation by q/2
  Dot roduct/1 -> inv1/1
  Product4/1 -> N_Uzonal(S)/1
  R/1 -> Product5/2
  inv/1 -> R/1
  inv1/1 -> inv/1, Gain1/1
  Constant/1 -> R/2
  To unit vector/1 -> Product1/2, Cross Product/1
  q(C->S)/1 -> " "/1, Vector rotation by q/1
  q(I->S)/1 -> " "/2
  " "/1 -> To unit vector/1
  Product2/1 -> Product1/1
  Product1/1 -> Cross Product/2
  I(C)/1 -> Product3/1
  Constant2/1 -> Product3/2
  Product3/1 -> Product2/1
  Constant1/1 -> Product2/2
  R_sc(I)/1 -> Dot roduct/2, Dot roduct/1, " "/3, Demux1/1
  Vector rotation by q/1 -> Product4/2
  Gain1/1 -> Product5/1
  Product5/1 -> Gain2/1
  Gain2/1 -> Product4/1

== system aausat3_lib/Dynamics and Kinematics/Spacecraft Dynamics ==
  Initial angular velocity W_i(S) : Inport
  Initial attitude q(I->S) : Inport  Port=2
  Controller frame  q(S->C) : Inport  Port=3
  Satellite Inertia I(C) : Inport  Port=4
  N_mt(S) : Inport  Port=5
  Disturbance N_dist(S) : Inport  Port=6
  Quaternion inverter : aausat3_lib/Math Utilities/Quaternion operations/Quaternion inverter
  Rotation of q1 by q1 : aausat3_lib/Math Utilities/Quaternion operations/Rotation of q1 by q2
  Rotation of q1 by q2 : aausat3_lib/Math Utilities/Quaternion operations/Rotation of q1 by q2
  S-Function : S-Function  FunctionName=scdynamics  EnableBusSupport=off
  Sum : Sum  Inputs=++|  SaturateOnIntegerOverflow=on
  Vector rotation by q : aausat3_lib/Math Utilities/Quaternion operations/Vector rotation by q
  Vector rotation by q1 : aausat3_lib/Math Utilities/Quaternion operations/Vector rotation by q
  Vector rotation by q3 : aausat3_lib/Math Utilities/Quaternion operations/Vector rotation by q
  w to q : aausat3_lib/Math Utilities/Quaternion operations/w to q
  Attitude q(I->S) : Outport
  Angular velocity W(S) : Outport  Port=2
  wires:
  Satellite Inertia I(C)/1 -> S-Function/3
  Sum/1 -> Vector rotation by q1/2
  Initial angular velocity W_i(S)/1 -> Vector rotation by q/2
  Controller frame  q(S->C)/1 -> Vector rotation by q/1, Rotation of q1 by q2/2, Vector rotation by q1/1, Quaternion inverter/1
  Initial attitude q(I->S)/1 -> Rotation of q1 by q2/1
  Vector rotation by q/1 -> S-Function/1
  Quaternion inverter/1 -> Vector rotation by q3/1, Rotation of q1 by q1/2
  Vector rotation by q3/1 -> Angular velocity W(S)/1
  Rotation of q1 by q2/1 -> w to q/2
  w to q/1 -> Rotation of q1 by q1/1
  S-Function/1 -> Vector rotation by q3/2, w to q/1
  Rotation of q1 by q1/1 -> Attitude q(I->S)/1
  N_mt(S)/1 -> Sum/1
  Disturbance N_dist(S)/1 -> Sum/2
  Vector rotation by q1/1 -> S-Function/2

== system aausat3_lib/Math Utilities/Projection Matrix ==
  n-vector : Inport
  Add : Sum  Inputs=+++
  Demux : Demux  Outputs=3
  Gain{1..6} (6 alike) : Gain  Gain=-1
  Math Funcion : Math  Operator=square  SaturateOnIntegerOverflow=on
  Math Function : Math  Operator=reciprocal  SaturateOnIntegerOverflow=on
  Math Function1 : Math  Operator=square  SaturateOnIntegerOverflow=on
  Math Function2 : Math  Operator=square  SaturateOnIntegerOverflow=on
  Mux : Mux  Inputs=9
  Product1 : Product  RndMeth=Zero
  Product2 : Product  RndMeth=Zero
  Product3 : Product  RndMeth=Zero
  Prouct : Product  RndMeth=Zero
  Reshape : Reshape  OutputDimensionality=Customize  OutputDimensions=[3,3]
  Sum : Sum  Inputs=|++
  Sum1 : Sum  Inputs=+|+
  Sum2 : Sum  Inputs=++|
  P matrix : Outport
  wires:
  Prouct/1 -> P matrix/1
  Reshape/1 -> Prouct/2
  Add/1 -> Math Function/1
  Math Function/1 -> Prouct/1
  n-vector/1 -> Demux/1
  Mux/1 -> Reshape/1
  Math Function1/1 -> Add/2, Sum/1, Sum2/2
  Math Function2/1 -> Add/3, Sum/2, Sum1/2
  Math Funcion/1 -> Add/1, Sum2/1, Sum1/1
  Sum1/1 -> Mux/5
  Sum2/1 -> Mux/9
  Sum/1 -> Mux/1
  Product3/1 -> Gain6/1, Gain4/1
  Product2/1 -> Gain5/1, Gain2/1
  Product1/1 -> Gain3/1, Gain1/1
  Gain6/1 -> Mux/8
  Gain5/1 -> Mux/7
  Gain4/1 -> Mux/6
  Gain3/1 -> Mux/4
  Gain2/1 -> Mux/3
  Gain1/1 -> Mux/2
  Demux/3 -> Product3/2, Math Function2/1, Product2/2
  Demux/2 -> Product3/1, Product1/2, Math Function1/1
  Demux/1 -> Product2/1, Product1/1, Math Funcion/1

== system aausat3_lib/Math Utilities/Quaternion operations ==
  Quaternion inverter : Subsystem
  Quaternion mulitiplication : S-Function  FunctionName=qmul  EnableBusSupport=off
  Rotation from q1 to q2 : Subsystem
  Rotation of q1 by q2 : Subsystem
  Vector rotation by q : Subsystem
  euler2quaternion : Subsystem
  quaternion composition : Subsystem
  quaternion decomposition : Subsystem
  quaternion2euler : Subsystem
  w to q : Subsystem

== system aausat3_lib/Math Utilities/Vector operations ==
  Cross Product : Subsystem
  To unit vector : Subsystem

== system aausat3_lib/Math Utilities/q_i_o calculator ==
  Vel_SC_I : Inport
  Pos_SC_I : Inport  Port=2
  Cross Product : aausat3_lib/Math Utilities/Vector operations/Cross Product  SystemSampleTime=-1
  Cross Product1 : aausat3_lib/Math Utilities/Vector operations/Cross Product  SystemSampleTime=-1
  Mux : Mux  Inputs=3
  To unit vector : aausat3_lib/Math Utilities/Vector operations/To unit vector  SystemSampleTime=-1
  To unit vector1 : aausat3_lib/Math Utilities/Vector operations/To unit vector  SystemSampleTime=-1
  inverse vector : Gain  Gain=-1
  quaternion calculator : MATLABFcn  Description=|  MATLABFcn=dcmatrix_and_q
      | Direction cosine matrix computation.                               
      | O1,O2,O3 are the three unit vectors representing the axes of the   
      | rotated coordinate system given in the reference coordinate system.
  q_I_O : Outport
  wires:
  Mux/1 -> quaternion calculator/1
  To unit vector1/1 -> inverse vector/1
  inverse vector/1 -> Cross Product/1, Mux/3, Cross Product1/2
  To unit vector/1 -> Cross Product/2
  Cross Product/1 -> Mux/2, Cross Product1/1
  Vel_SC_I/1 -> To unit vector/1
  Pos_SC_I/1 -> To unit vector1/1
  quaternion calculator/1 -> q_I_O/1
  Cross Product1/1 -> Mux/1

== system aausat3_lib/On-board Software/Ephemeris ==
  Time t(JD) : Inport  SampleTime=1/f_sample
  ECI->ECEF quaternion : Subsystem
  Sun Position : Subsystem
  Sun Position R_s(I) : Outport
  Earth Rotation q(I->E) : Outport  Port=2
  wires:
  ECI->ECEF quaternion/1(q(I->E)) -> Earth Rotation q(I->E)/1  "q(I -> E)"
  Time t(JD)/1 -> ECI->ECEF quaternion/1(t(JD)), Sun Position/1(t(JD))
  Sun Position/1(R_s(I)) -> Sun Position R_s(I)/1  "R_s(I)"

== system aausat3_lib/On-board Software/Orbit and Magnetic field models ==
  Earth rotation q(I->E) : Inport
  Sun position R_s(I) : Inport  Port=2
  Initial time ti(JD) : Inport  Port=3
  TLE : Inport  Port=4
  (IGRF) Magnetic field : Subsystem  TreatAsAtomicUnit=on
  Custom time : Subsystem  TreatAsAtomicUnit=on
  Eclipse model : Subsystem  mask{r_e=r_e, enable=off, theta_e=theta_e}
      mask prompts: r_e "Radius of Earth [m]"; enable "Enable max angle"; theta_e "Max. angle of theta [deg] (eclipse: theta > r_earth/norm(R_SA))"
      mask Display: fprintf('1=true,\n 0=false')
  Gain : Gain  Gain=1e-4
  Quaternion inverter : Subsystem
  SGP4 position : Subsystem  TreatAsAtomicUnit=on
  Terminator : Terminator
  Vector rotation by q : Subsystem
  enable SGP4 : Constant  Value=enable_sgp4
  enable eclipse : Constant  Value=enable_eclipse
  enable time : Constant  Value=enable_custom_time
  enable?1 : Constant  Value=enable_IGRF
  initial time : Subsystem
  Mag [Tesla] B(I) : Outport
  Simulation time t(JD) : Outport  Port=2
  "Eclipse: 1=true, 0=false" : Outport  Port=3  PortDimensions=1
  wires:
  Initial time ti(JD)/1 -> initial time/1(Initial time in (JD))
  initial time/1(Initial time out (JD)) -> Custom time/1(Initial time ti(JD))
  TLE/1 -> initial time/2(TLE), SGP4 position/2(TLE)
  enable eclipse/1 -> Eclipse model/Enable
  Gain/1 -> Mag [Tesla] B(I)/1
  (IGRF) Magnetic field/1(Magnetic field vector B(E)) -> Vector rotation by q/2(V)
  SGP4 position/1(Position (I)) -> Eclipse model/2(Satellite (I)), (IGRF) Magnetic field/1(Spacecraft position R_sc(I))
  enable SGP4/1 -> SGP4 position/Enable
  Earth rotation q(I->E)/1 -> Quaternion inverter/1(q), (IGRF) Magnetic field/2(Earth rotation q(I->E))
  Custom time/1(Simulation time t(JD)) -> SGP4 position/1(JD), Simulation time t(JD)/1
  enable time/1 -> Custom time/Enable
  Quaternion inverter/1(q^-1) -> Vector rotation by q/1(q)
  Vector rotation by q/1(q'Vq) -> Gain/1
  enable?1/1 -> (IGRF) Magnetic field/Enable
  Eclipse model/1(Eclipse) -> "Eclipse: 1=true, 0=false"/1
  Sun position R_s(I)/1 -> Eclipse model/1(Sun vector (I))
  SGP4 position/2(Velocity (I)) -> Terminator/1

== system aausat3_lib/Orbit and Ephemeris/(IGRF) Magnetic field ==
  Spacecraft position R_sc(I) : Inport
  Earth rotation q(I->E) : Inport  Port=2
  Enable : EnablePort
  Magnetic field model : Subsystem
  T->Gauss : Gain  Gain=1e4  SaturateOnIntegerOverflow=on  OutDataTypeStr=Inherit: Same as input  ParamDataTypeStr=Inherit: Same as input
  Vector rotation by q : aausat3_lib/Math Utilities/Quaternion operations/Vector rotation by q  SystemSampleTime=-1
  Magnetic field vector B(E) : Outport
  wires:
  T->Gauss/1 -> Magnetic field vector B(E)/1
  Magnetic field model/1(B(E)) -> T->Gauss/1  "B(I / E)"
  Vector rotation by q/1 -> Magnetic field model/1(R_sc(E))
  Earth rotation q(I->E)/1 -> Vector rotation by q/1
  Spacecraft position R_sc(I)/1 -> Vector rotation by q/2

== system aausat3_lib/Orbit and Ephemeris/Albedo ==
  Sunlight vector(I) : Inport
  Nadir vector (I) : Inport  Port=2
  q(I>E) : Inport  Port=3
  Enable : EnablePort
  Earth Albedo Model : Subsystem  TreatAsAtomicUnit=on  mask(Earth Albedo Model){refldata=refldata, redfac=redfac, Ts=Ts}
      mask prompts: refldata "Reflectivity Data (REFL Struct):"; redfac "Reduction factor:"; Ts "Sample Time (-1 for inherited):"
      mask help: Calculcates the Earth albedo from satellite and Sun positions and static reflectivity data.
      mask init:
      | global sy;
      | global sx;
      | sy = floor(180/redfac);
      | sx = floor(288/redfac);
      mask Help:
      | <b>Input</b><br>
      | Sat: Vector to satellite in ECEF [m].<br>
      | Sun: Vector to the Sun in ECEF [m].<p>
      | <b>Parameters</b><br>
      | Reflectivity Data (REFL Struct): TOMS Reflectivity data [E.U].<br>
      | Reduction factor: Reduce data resolution by this factor.<br>
      | Sample Time (-1 for inherited): Sample Time [s]. The block cannot inherit continuous sample time.<br>
      | Enable: Enable or disable albedo calculation.<p>
      | <b>Output</b><br>
      | Albedo: Fraction of solar irradiance received on the satellite. The incoming solar irradiance is 1366.5 W/m^2.<p>
  Vector rotation by q : aausat3_lib/Math Utilities/Quaternion operations/Vector rotation by q  SystemSampleTime=-1
  Vector rotation by q1 : aausat3_lib/Math Utilities/Quaternion operations/Vector rotation by q  SystemSampleTime=-1
  Reflectivity matrix : Outport
  wires:
  Vector rotation by q/1 -> Earth Albedo Model/1(r_sat_ecef)
  Vector rotation by q1/1 -> Earth Albedo Model/2(r_sun_ecef)
  Earth Albedo Model/1(a) -> Reflectivity matrix/1
  Nadir vector (I)/1 -> Vector rotation by q/2
  q(I>E)/1 -> Vector rotation by q/1, Vector rotation by q1/1
  Sunlight vector(I)/1 -> Vector rotation by q1/2

== system aausat3_lib/Orbit and Ephemeris/Custom time ==
  Initial time ti(JD) : Inport
  Enable : EnablePort
  Clock : Clock
  Sec2Day : Gain  Gain=1/86400  SaturateOnIntegerOverflow=on  OutDataTypeStr=Inherit: Same as input  ParamDataTypeStr=Inherit: Same as input
  Sum : Sum  Inputs=|++
  Simulation time t(JD) : Outport
  wires:
  Sum/1 -> Simulation time t(JD)/1
  Clock/1 -> Sec2Day/1
  Sec2Day/1 -> Sum/2
  Initial time ti(JD)/1 -> Sum/1

== system aausat3_lib/Orbit and Ephemeris/ECI->ECEF quaternion ==
  t(JD) : Inport
  MATLAB Function : MATLAB Function  TreatAsAtomicUnit=on
  q(I->E) : Outport
  wires:
  t(JD)/1 -> MATLAB Function/1(u)
  MATLAB Function/1(y) -> q(I->E)/1

== system aausat3_lib/Orbit and Ephemeris/Eclipse model ==
  note: theta_e
  Sun vector (I) : Inport
  Satellite (I) : Inport  Port=2
  Enable : EnablePort
  Constant : Constant  Value=pi
  Constant1 : Constant  Value=enable
  Divide : Product  Inputs=*/
  Dot Product : DotProduct  InputSameDT=on  OutDataTypeStr=Inherit: Inherit via internal rule
  Dot Product1 : DotProduct  InputSameDT=on  OutDataTypeStr=Inherit: Inherit via internal rule
  Earth radius : Constant  Value=r_e
  False : Constant  Value=0
  Math Function : Math  Operator=sqrt  SaturateOnIntegerOverflow=on
  Max angle : Constant  Value=theta_e/180*pi
  Sum : Sum  Inputs=-+|
  Sum1 : Sum  Inputs=+-|
  Switch : Switch
  Switch1 : Switch  Criteria=u2 > Threshold
  To unit vector : aausat3_lib/Math Utilities/Vector operations/To unit vector  SystemSampleTime=-1
  To unit vector1 : aausat3_lib/Math Utilities/Vector operations/To unit vector  SystemSampleTime=-1
  Trigonometric Function : Trigonometry  Operator=asin
  Trigonometric Function1 : Trigonometry  Operator=acos
  True : Constant
  Eclipse : Outport  PortDimensions=1
  wires:
  Dot Product1/1 -> Math Function/1
  Trigonometric Function/1 -> Switch1/3
  Switch1/1 -> Sum1/2
  Switch/1 -> Eclipse/1
  False/1 -> Switch/1
  True/1 -> Switch/3
  Sum1/1 -> Switch/2
  Sum/1 -> Sum1/1  "theta"
  Constant/1 -> Sum/2
  Trigonometric Function1/1 -> Sum/1
  Divide/1 -> Trigonometric Function/1
  Math Function/1 -> Divide/2
  Earth radius/1 -> Divide/1
  Dot Product/1 -> Trigonometric Function1/1
  To unit vector1/1 -> Dot Product/2
  To unit vector/1 -> Dot Product/1
  Satellite (I)/1 -> Dot Product1/2, Dot Product1/1, To unit vector1/1
  Sun vector (I)/1 -> To unit vector/1
  Constant1/1 -> Switch1/2
  Max angle/1 -> Switch1/1

== system aausat3_lib/Orbit and Ephemeris/Ephemeris ==
  Time t(JD) : Inport
  ECI->ECEF quaternion : aausat3_lib/Orbit and Ephemeris/ECI->ECEF quaternion
  Moon Position : Subsystem
  Sun Position : Subsystem
  Moon position R_m(I) : Outport
  Sun Position R_s(I) : Outport  Port=2
  Earth Rotation q(I->E) : Outport  Port=3
  wires:
  Sun Position/1(R_s(I)) -> Sun Position R_s(I)/1  "R_s(I)"
  Moon Position/1(R_m(I)) -> Moon position R_m(I)/1  "R_m(I)"
  Time t(JD)/1 -> Moon Position/1(t(JD)1), ECI->ECEF quaternion/1, Sun Position/1(t(JD))  "t"
  ECI->ECEF quaternion/1 -> Earth Rotation q(I->E)/1  "q(I -> E)"

== system aausat3_lib/Orbit and Ephemeris/Magnetic field model ==
  R_sc(E) : Inport
  S-Function : S-Function  FunctionName=igrfS  Parameters=2002,10  EnableBusSupport=off
  B(E) : Outport
  wires:
  S-Function/1 -> B(E)/1
  R_sc(E)/1 -> S-Function/1

== system aausat3_lib/Orbit and Ephemeris/Orbit and Magnetic field models ==
  Earth rotation q(I->E) : Inport
  Sun position R_s(I) : Inport  Port=2
  Initial time ti(JD) : Inport  Port=3
  TLE : Inport  Port=4
  (IGRF) Magnetic field : aausat3_lib/Orbit and Ephemeris/(IGRF) Magnetic field
  Custom time : aausat3_lib/Orbit and Ephemeris/Custom time
  Eclipse model : aausat3_lib/Orbit and Ephemeris/Eclipse model  r_e=r_e  enable=off  theta_e=theta_e
  Gain : Gain  Gain=1e-4
  Quaternion inverter : aausat3_lib/Math Utilities/Quaternion operations/Quaternion inverter
  SGP4 position : aausat3_lib/Orbit and Ephemeris/SGP4 position
  Vector rotation by q : aausat3_lib/Math Utilities/Quaternion operations/Vector rotation by q
  enable SGP4 : Constant  Value=enable_sgp4
  enable eclipse : Constant  Value=enable_eclipse
  enable time : Constant  Value=enable_custom_time
  enable?1 : Constant  Value=enable_IGRF
  initial time : Subsystem
  Mag [Tesla] B(I) : Outport
  Spacecraft velocity V (I) : Outport  Port=2
  Spacecraft position R (I) : Outport  Port=3
  Simulation time t(JD) : Outport  Port=4
  "Eclipse: 1=true, 0=false" : Outport  Port=5  PortDimensions=1
  wires:
  Eclipse model/1 -> "Eclipse: 1=true, 0=false"/1
  enable?1/1 -> (IGRF) Magnetic field/Enable
  Vector rotation by q/1 -> Gain/1
  Quaternion inverter/1 -> Vector rotation by q/1
  enable time/1 -> Custom time/Enable
  Custom time/1 -> Simulation time t(JD)/1, SGP4 position/1
  Sun position R_s(I)/1 -> Eclipse model/1
  Earth rotation q(I->E)/1 -> (IGRF) Magnetic field/2, Quaternion inverter/1
  enable SGP4/1 -> SGP4 position/Enable
  SGP4 position/1 -> (IGRF) Magnetic field/1, Eclipse model/2, Spacecraft position R (I)/1
  SGP4 position/2 -> Spacecraft velocity V (I)/1
  (IGRF) Magnetic field/1 -> Vector rotation by q/2
  Gain/1 -> Mag [Tesla] B(I)/1
  enable eclipse/1 -> Eclipse model/Enable
  TLE/1 -> SGP4 position/2, initial time/2(TLE)
  initial time/1(Initial time out (JD)) -> Custom time/1
  Initial time ti(JD)/1 -> initial time/1(Initial time in (JD))
